simulink model "findUnitVec_th"  (R2018b)
settings: Solver=VariableStepAuto  StartTime=0.0  StopTime=0  RelTol=1e-3
libraries: findUnitVectors_ul x1
settings Model: Creator=asiddiq2  LastModifiedBy=asiddiq2

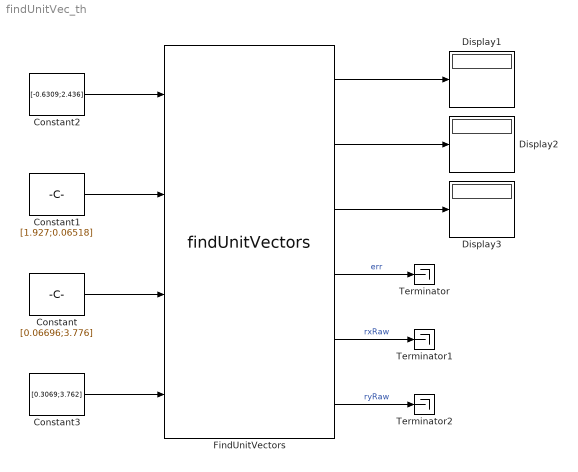
== system findUnitVec_th ==
  Constant : Constant  Value=[0.06696;3.776]
  Constant1 : Constant  Value=[1.927;0.06518]
  Constant2 : Constant  Value=[-0.6309;2.436]
  Constant3 : Constant  Value=[0.3069;3.762]
  Display1 : Display
  Display2 : Display
  Display3 : Display
  FindUnitVectors : findUnitVectors_ul/findUnitVectors  sideSeparation_cm=params.sideDotSepDist_cm.Value  bottomASeparation_cm=params.botADotSepDist_cm.Value  bottomBSeparation_cm=params.botBDotSepDist_cm.Value  topSeparation_cm=params.topDotSepDist_cm.Value  DSB=[0 -.5 -.5 0;0 0 0 1;-1 0 0 0]  DBL=[-1 0 0 0;0 0.5 0 0.5; 0 0 -1 0]
  Terminator : Terminator
  Terminator1 : Terminator
  Terminator2 : Terminator
  wires:
  Constant3/1 -> FindUnitVectors/4
  FindUnitVectors/1 -> Display1/1
  FindUnitVectors/2 -> Display2/1
  FindUnitVectors/3 -> Display3/1
  Constant/1 -> FindUnitVectors/3
  Constant2/1 -> FindUnitVectors/1
  Constant1/1 -> FindUnitVectors/2
  FindUnitVectors/6 -> Terminator2/1  "ryRaw"
  FindUnitVectors/5 -> Terminator1/1  "rxRaw"
  FindUnitVectors/4 -> Terminator/1  "err"
